simulink model "WayPoint"  (R2019a)
settings: Solver=FixedStepAuto  StartTime=0.0  StopTime=inf  FixedStep=0.05  RelTol=1e-3
undefined symbols (not defined in the file): Angular, Linear
libraries: robotlib x3, simulink x1
settings Model: Creator=user  LastModifiedBy=user
settings OptimizationCC: EnhancedBackFolding=on  PassReuseOutputArgsAs=Individual arguments  MaxStackSize=64  OptimizeBlockOrder=speed  DifferentSizesBufferReuse=on  OptimizationCustomize=off
settings DebuggingCC: ParameterTunabilityLossMsg=error
settings HardwareCC: ProdBitPerPointer=32  ProdBitPerSizeT=32  ProdBitPerPtrDiffT=32  ProdLargestAtomicFloat=None  ProdIntDivRoundTo=Undefined  ProdEndianess=Unspecified  ProdWordSize=32  ProdHWDeviceType=Generic->Unspecified (assume 32-bit Generic)
settings SFSimCC: MATLABDynamicMemAlloc=off
settings RTWCC: SystemTargetFile=ert.tlc  HardwareBoard=Robot Operating System (ROS)  TLCOptions="-aInlineSetEventsForThisBaseRateFcn=TLC_FALSE -aSuppressMultiTaskScheduler=TLC_FALSE  -aRateBasedStepFcn=0"  TemplateMakefile=ert_default_tmf  GenerateReport=on  Toolchain=Catkin  IncludeHyperlinkInReport=on  LaunchReport=on  TargetLang=C++  GenerateTraceInfo=on  GenerateTraceReport=on  GenerateTraceReportSl=on  GenerateTraceReportSf=on  GenerateTraceReportEml=on
settings CodeAppCC: ForceParamTrailComments=on  IgnoreCustomStorageClasses=off  OperatorAnnotations=on  SimulinkDataObjDesc=on  SFDataObjDesc=on  InsertBlockDesc=on

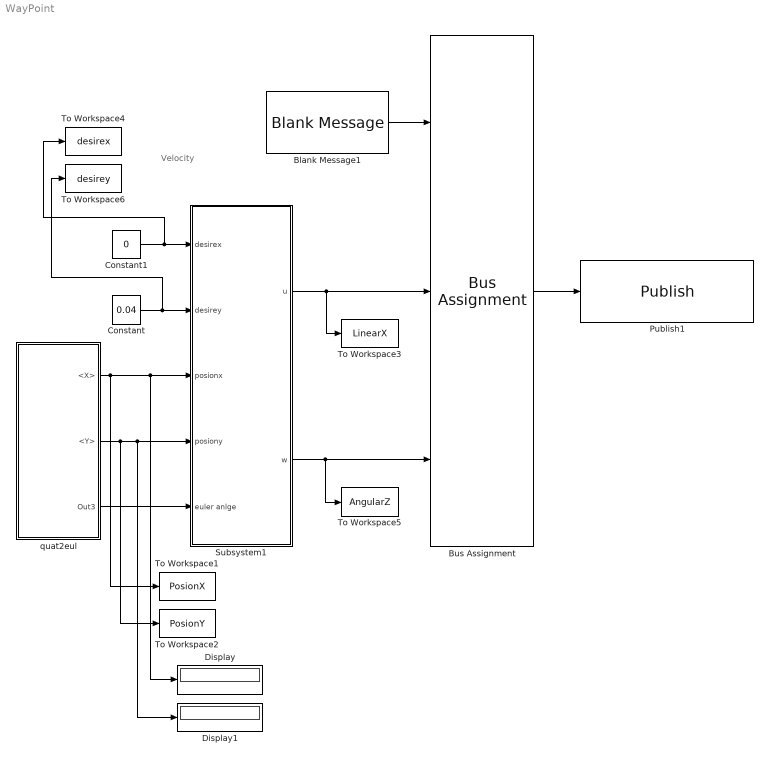
== system WayPoint ==
  note: Velocity
  Blank Message1 : robotlib/Blank Message  messageClass=Message  entityType=geometry_msgs/Twist  messageType=geometry_msgs/Twist  SampleTime=inf
      settings: SourceProductBaseCode=RO
  Bus Assignment : BusAssignment  AssignedSignals=Linear.X,Angular.Z
  Constant : Constant  Value=0.04
  Constant1 : Constant  Value=0
  Display : Display
  Display1 : Display
  Publish1 : robotlib/Publish  topicSource=Select from ROS network  topic=/cmd_vel  messageType=geometry_msgs/Twist  messageQueueLength=1
      settings: SourceProductBaseCode=RO
  Subsystem1 : Subsystem
  To Workspace1 : ToWorkspace  VariableName=PosionX  SampleTime=-1
      settings: Save2DSignal=2-D array (concatenate along first dimension)
  To Workspace2 : ToWorkspace  VariableName=PosionY  SampleTime=-1
      settings: Save2DSignal=2-D array (concatenate along first dimension)
  To Workspace3 : ToWorkspace  VariableName=LinearX  SampleTime=-1
      settings: Save2DSignal=2-D array (concatenate along first dimension)
  To Workspace4 : ToWorkspace  VariableName=desirex  SampleTime=-1
      settings: Save2DSignal=2-D array (concatenate along first dimension)
  To Workspace5 : ToWorkspace  VariableName=AngularZ  SampleTime=-1
      settings: Save2DSignal=2-D array (concatenate along first dimension)
  To Workspace6 : ToWorkspace  VariableName=desirey  SampleTime=-1
      settings: Save2DSignal=2-D array (concatenate along first dimension)
  quat2eul : Subsystem
  wires:
  Blank Message1/1 -> Bus Assignment/1
  Bus Assignment/1 -> Publish1/1
  Subsystem1/1(u) -> To Workspace3/1, Bus Assignment/2
  Subsystem1/2(w) -> To Workspace5/1, Bus Assignment/3
  quat2eul/1(<X>) -> To Workspace1/1, Display/1, Subsystem1/3(posionx)
  quat2eul/2(<Y>) -> To Workspace2/1, Display1/1, Subsystem1/4(posiony)
  quat2eul/3(Out3) -> Subsystem1/5(euler anlge)
  Constant/1 -> To Workspace6/1, Subsystem1/2(desirey)
  Constant1/1 -> To Workspace4/1, Subsystem1/1(desirex)

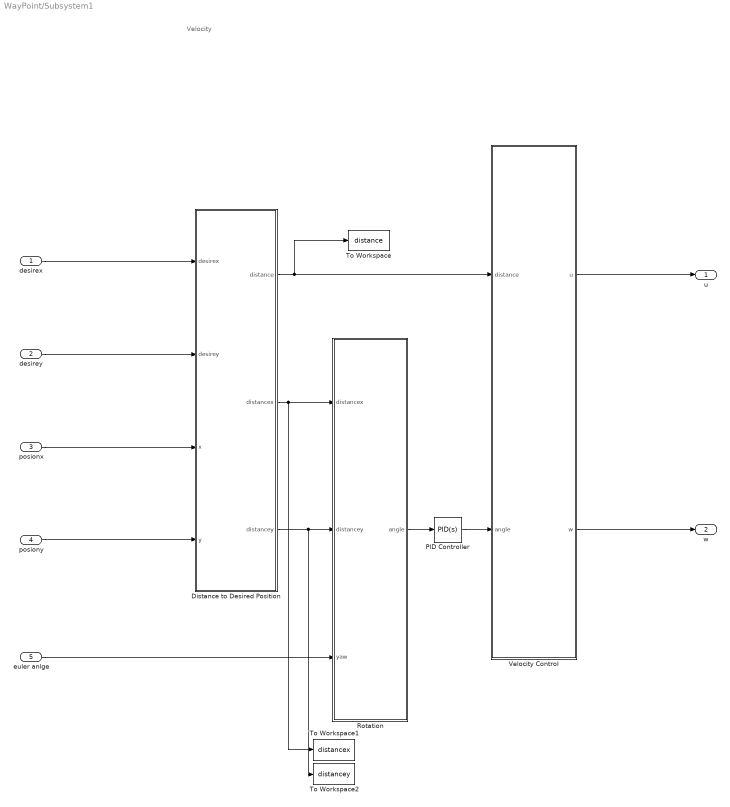
== system WayPoint/Subsystem1 ==
  note: Velocity
  desirex : Inport
  desirey : Inport  Port=2
  posionx : Inport  Port=3
  posiony : Inport  Port=4
  euler anlge : Inport  Port=5
  Distance to Desired Position : MATLAB Function  TreatAsAtomicUnit=on
  PID Controller : simulink/Continuous/PID Controller  Controller=PID  Form=Parallel  TimeDomain=Continuous-time  SampleTime=-1  IntegratorMethod=Forward Euler  FilterMethod=Forward Euler  ControllerParametersSource=internal  P=1.1  I=0  D=0  UseFilter=on  N=100  TunerSelectOption=Transfer Function Based (PID Tuner App)  InitialConditionSource=internal  InitialConditionForIntegrator=0  InitialConditionForFilter=0  DifferentiatorICPrevScaledInput=0  ExternalReset=none  TrackingMode=off  Kt=1  LimitOutput=off  UpperSaturationLimit=inf  LowerSaturationLimit=-inf  LinearizeAsGain=on  AntiWindupMode=none  Kb=1  POutMin=[]  POutMax=[]  IOutMin=[]  IOutMax=[]  DOutMin=[]  DOutMax=[]  NOutMin=[]  NOutMax=[]  SumOutMin=[]  SumOutMax=[]  SaturationOutMin=[]  SaturationOutMax=[]  PParamMin=[]  PParamMax=[]  IParamMin=[]  IParamMax=[]  DParamMin=[]  DParamMax=[]  NParamMin=[]  NParamMax=[]  KbParamMin=[]  KbParamMax=[]  KtParamMin=[]  KtParamMax=[]  KbOutMin=[]  KbOutMax=[]  KtOutMin=[]  KtOutMax=[]  IntegratorOutMin=[]  IntegratorOutMax=[]  FilterOutMin=[]  FilterOutMax=[]  SumI1OutMin=[]  SumI1OutMax=[]  SumI2OutMin=[]  SumI2OutMax=[]  SumI3OutMin=[]  SumI3OutMax=[]  SumI4OutMin=[]  SumI4OutMax=[]  SumDOutMin=[]  SumDOutMax=[]  DifferentiatorOutMin=[]  DifferentiatorOutMax=[]  FilterDiffOutCoefMin=[]  FilterDiffOutCoefMax=[]  ReciprocalOutMin=[]  ReciprocalOutMax=[]  SumDenOutMin=[]  SumDenOutMax=[]  SumNumOutMin=[]  SumNumOutMax=[]  DivideOutMin=[]  DivideOutMax=[]  IntegratorContinuousStateAttributes=''  IntegratorStateMustResolveToSignalObject=off  IntegratorRTWStateStorageClass=Auto  FilterContinuousStateAttributes=''  FilterStateMustResolveToSignalObject=off  FilterRTWStateStorageClass=Auto  ParallelPVariant=InternalParameters  IdealPVariant=Disabled  IVariant=InternalParameters  DVariant=InternalParameters  IntegratorVariant=Continuous  SatVariant=Disabled  AWVariant=Passthrough  PCopyVariant=Disabled  TRVariant=Disabled  FdbkBlocksVariant=Forward  IdealPFdbkVariant=Disabled  SatFdbkVariant=Disabled  DerivativeFilterVariant=ContFilter  NVariant=InternalParameters  NCopyVariant=Disabled  FilterICVariant=InternalICsFilter  IntegratorICVariant=InternalICs  ExternalResetVariant=Disabled  TRSumVariant=Passthrough  SumFdbkVariant=Disabled  SumVariant=Sum_PID
  Rotation : MATLAB Function  TreatAsAtomicUnit=on
  To Workspace : ToWorkspace  VariableName=distance  SampleTime=-1
      settings: Save2DSignal=2-D array (concatenate along first dimension)
  To Workspace1 : ToWorkspace  VariableName=distancex  SampleTime=-1
      settings: Save2DSignal=2-D array (concatenate along first dimension)
  To Workspace2 : ToWorkspace  VariableName=distancey  SampleTime=-1
      settings: Save2DSignal=2-D array (concatenate along first dimension)
  Velocity Control : MATLAB Function  TreatAsAtomicUnit=on
  u : Outport
  w : Outport  Port=2
  wires:
  desirex/1 -> Distance to Desired Position/1(desirex)
  desirey/1 -> Distance to Desired Position/2(desirey)
  Distance to Desired Position/2(distancex) -> To Workspace1/1, Rotation/1(distancex)
  Velocity Control/2(w) -> w/1
  posionx/1 -> Distance to Desired Position/3(x)
  euler anlge/1 -> Rotation/3(yaw)
  posiony/1 -> Distance to Desired Position/4(y)
  Rotation/1(angle) -> PID Controller/1
  PID Controller/1 -> Velocity Control/2(angle)
  Distance to Desired Position/3(distancey) -> To Workspace2/1, Rotation/2(distancey)
  Distance to Desired Position/1(distance) -> Velocity Control/1(distance), To Workspace/1
  Velocity Control/1(u) -> u/1

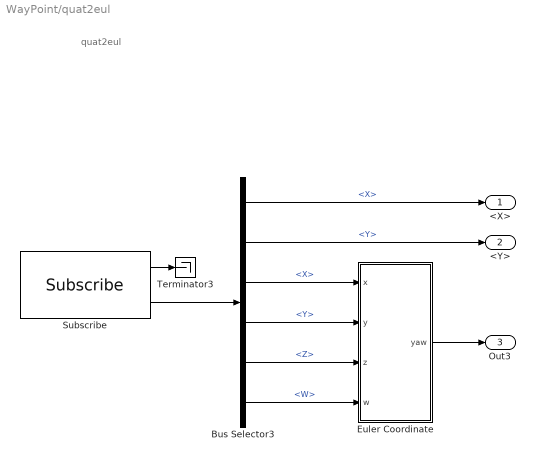
== system WayPoint/quat2eul ==
  note: quat2eul
  Bus Selector3 : BusSelector  OutputSignals=Pose.Pose.Position.X,Pose.Pose.Position.Y,Pose.Pose.Orientation.X,Pose.Pose.Orientation.Y,Pose.Pose.Orientation.Z,Pose.Pose.Orientation.W
  Euler Coordinate : MATLAB Function  TreatAsAtomicUnit=on
  Subscribe : robotlib/Subscribe  topicSource=Select from ROS network  topic=/odom  messageType=nav_msgs/Odometry  sampleTime=-1  messageQueueLength=1
      settings: SourceProductBaseCode=RO
  Terminator3 : Terminator
  <X> : Outport
  <Y> : Outport  Port=2
  Out3 : Outport  Port=3
  wires:
  Euler Coordinate/1(yaw) -> Out3/1
  Bus Selector3/5 -> Euler Coordinate/3(z)  "<Z>"
  Bus Selector3/6 -> Euler Coordinate/4(w)  "<W>"
  Subscribe/1 -> Terminator3/1
  Bus Selector3/3 -> Euler Coordinate/1(x)  "<X>"
  Subscribe/2 -> Bus Selector3/1
  Bus Selector3/4 -> Euler Coordinate/2(y)  "<Y>"
  Bus Selector3/2 -> <Y>/1  "<Y>"
  Bus Selector3/1 -> <X>/1  "<X>"

== matlab function WayPoint/quat2eul/Euler Coordinate ==
  data: x input; yaw output; y input; z input; w input
function yaw = quat2eul(x,y,z,w)

eul = quat2eul([w,x,y,z]);
yaw = eul(1);

end

== matlab function WayPoint/Subsystem1/Velocity Control ==
  data: distance input; u output; angle input; w output
function [u,w] = velocity(distance,angle)

if (angle <= 0.05) && (angle >= -0.05)
    u = 0.07;
    if (distance <= 0.003)
        u = 0;
    end
else
    u = 0;
end

w = angle;

== matlab function WayPoint/Subsystem1/Rotation ==
  data: distancex input; angle output; distancey input; yaw input
function angle = angle(distancex,distancey,yaw)

desireangle = atan2(distancey,distancex);
u = desireangle - yaw;
angle =  atan2(sin(u),cos(u));

== matlab function WayPoint/Subsystem1/Distance to Desired Position ==
  data: distance output; desirex input; distancex output; desirey input; x input; y input; distancey output
function [distance,distancex,distancey] = distance(desirex,desirey,x,y)



distancex = desirex - x;
distancey = desirey - y;
distance = sqrt(distancex^2 + distancey^2);
